simulink model "AccTarSel"  (R2018b)
settings: Solver=FixedStepDiscrete  StartTime=0.0  StopTime=inf  FixedStep=0.01  RelTol=1e-3
PostLoadFcn:
  | if any(exist('dsrtsu_mdlpostloadfcn', 'file') ~= 0), dsrtsu_mdlpostloadfcn('Execute', bdroot); end
values from neighbouring files (symbols this model uses):
  P_adtMaxBDC = 1.0    [AccTarSel.sldd]
  P_aFOCApproachIntpAcitve = -0.6    [AccTarSel.sldd]
  P_aFOCApproachIntpEnsure = -1.8    [AccTarSel.sldd]
  P_CutInEnable = 1.0    [AccTarSel.sldd]
  P_dAimMin = 4.5    [AccTarSel.sldd]
  P_dAimMinAVP = 1.5    [AccTarSel.sldd]
  P_dObjDrvOffMax = 5.0    [AccTarSel.sldd]
  P_dObjDrvOffMin = 3.0    [AccTarSel.sldd]
  P_dObjLowHystDecToStop = 4.5    [AccTarSel.sldd]
  P_dObjLowHystDecToStopAVP = 1.5    [AccTarSel.sldd]
  P_dObjUpperHystDecToStop = 5.0    [AccTarSel.sldd]
  P_dResMax = 5.0    [AccTarSel.sldd]
  P_dStandStill = 3.0    [AccTarSel.sldd]
  P_dStandStillMin = 2.0    [AccTarSel.sldd]
  P_dvarYMax4PO = 1.0    [AccTarSel.sldd]
  P_dyCutInThres = 3.6    [AccTarSel.sldd]
  P_facBDCInit = 0.7    [AccTarSel.sldd]
  P_facBDCIterCalc = 0.8    [AccTarSel.sldd]
  P_facFOCNegDiff = 0.3    [AccTarSel.sldd]
  P_facFOCPosDiff = 0.2    [AccTarSel.sldd]
  P_kapHystThres = 0.0005    [AccTarSel.sldd]
  P_PlausIntegDisable = 0.0    [AccTarSel.sldd]
  P_plausMin4PO = 0.5    [AccTarSel.sldd]
  P_probExistMin4PO = 0.8    [AccTarSel.sldd]
  P_StandObjEnable = 0.0    [AccTarSel.sldd]
  P_tAxTrackNegLower = 0.3    [AccTarSel.sldd]
  P_tAxTrackNegUpper = 0.6    [AccTarSel.sldd]
  P_tAxTrackPosLower = 1.0    [AccTarSel.sldd]
  P_tAxTrackPosUpper = 2.0    [AccTarSel.sldd]
  P_tBDCStartFilt = 0.2    [AccTarSel.sldd]
  P_tCSC = 3.5    [AccTarSel.sldd]
  P_tCurvFilt = 0.2    [AccTarSel.sldd]
  P_tCutInFilt = 0.5    [AccTarSel.sldd]
  P_tFiltAxAbsPONegFast = 0.1    [AccTarSel.sldd]
  P_tFiltAxAbsPONegSlow = 0.4    [AccTarSel.sldd]
  P_tFiltAxAbsPOPosFast = 1.2    [AccTarSel.sldd]
  P_tFiltAxAbsPOPosSlow = 2.0    [AccTarSel.sldd]
  P_tFiltAxAbsPOStand = 2.0    [AccTarSel.sldd]
  P_tFiltDAim = 0.1    [AccTarSel.sldd]
  P_tFiltDsd = 0.1    [AccTarSel.sldd]
  P_tFiltSpdLim = 3.0    [AccTarSel.sldd]
  P_tFiltVxAxPOFast = 0.15    [AccTarSel.sldd]
  P_tFiltVxAxPOSlow = 0.25    [AccTarSel.sldd]
  P_tFOCStatAccelFast = 4.0    [AccTarSel.sldd]
  P_tFOCStatAccelSlow = 3.5    [AccTarSel.sldd]
  P_tFOCStatDecelFast = 4.0    [AccTarSel.sldd]
  P_tFOCStatDecelSlow = 3.2    [AccTarSel.sldd]
  P_tMinDrvPhase = 2.0    [AccTarSel.sldd]
  P_tPredObjLeav = 1.2    [AccTarSel.sldd]
  P_tRollingFilt = 0.5    [AccTarSel.sldd]
  P_tRollingFinFilt = 1.0    [AccTarSel.sldd]
  P_tSSCNeg = 4.5    [AccTarSel.sldd]
  P_tSSCPos = 5.5    [AccTarSel.sldd]
  P_tToStop = 5.0    [AccTarSel.sldd]
  P_tToStopInBDC = 6.0    [AccTarSel.sldd]
  P_tToStopTrig = 4.0    [AccTarSel.sldd]
  P_vEgoDecToStop = 3.0    [AccTarSel.sldd]
  P_vEgoLowBDC = 4.0    [AccTarSel.sldd]
  P_vFOCNegDiff = 4.0    [AccTarSel.sldd]
  P_vFOCPosDiff = 5.0    [AccTarSel.sldd]
  P_vFOCStationaryFast = 15.0    [AccTarSel.sldd]
  P_vFOCStationarySlow = 5.0    [AccTarSel.sldd]
  P_vObjDrvOff = 0.5    [AccTarSel.sldd]
  P_vObjLowHystDecToStop = 0.5    [AccTarSel.sldd]
  P_vObjNoStop = 1.0    [AccTarSel.sldd]
  P_vObjReCalc = 1.0    [AccTarSel.sldd]
  P_vObjStop = 0.3    [AccTarSel.sldd]
  P_vObjUpperHystDecToStop = 0.8    [AccTarSel.sldd]
  P_vStandStill = 0.3    [AccTarSel.sldd]
  P_vStandStillHyst = 0.3    [AccTarSel.sldd]
  P_vyCutInThres = 0.5    [AccTarSel.sldd]
libraries: simulink x21, LPFilter x12
(part 4 of 11)

== system AccTarSel/ACC_dTarSet1/If Action Subsystem2 ==
  In1 : Inport
  Action Port : ActionPort  ActionType=else
  Out1 : Outport
  wires:
  In1/1 -> Out1/1

== system AccTarSel/ACC_dTarSet1/Subsystem ==
  ACCState : Inport
  Constant : Constant  Value=2  OutDataTypeStr=single
  Equal1 : RelationalOperator  Operator===  OutDataTypeStr=boolean  RndMeth=Simplest
  PreCon : Outport
  wires:
  Constant/1 -> Equal1/2
  ACCState/1 -> Equal1/1
  Equal1/1 -> PreCon/1

== system AccTarSel/AVP_Simu/AVP_Activate ==
  Action Port : ActionPort  ActionType=then
  Constant : Constant  OutDataTypeStr=single
  Out1 : Outport
  wires:
  Constant/1 -> Out1/1

== system AccTarSel/AVP_Simu/AVP_Deactivate ==
  Action Port : ActionPort  ActionType=elseif
  Constant : Constant  Value=0  OutDataTypeStr=single
  Out1 : Outport
  wires:
  Constant/1 -> Out1/1

== system AccTarSel/AVP_Simu/Hold ==
  AVP_ActiveK1 : Inport
  Action Port : ActionPort  ActionType=else
  Out1 : Outport
  wires:
  AVP_ActiveK1/1 -> Out1/1

== system AccTarSel/AVP_Simu/calcAVPInfo ==
  note: 00: Invalid
      | 01:Parking In
      | 02:Parking Out
      | 03:Stop
  AVP_Info : Inport
  egoInfo : Inport  Port=2
  SYS_Info : Inport  Port=3
  Bus Creator : BusCreator  Inputs=7  OutDataTypeStr=Bus: AVP_OUTPUT_ST  NonVirtualBus=on
      settings: InheritFromInputs=off
  Bus Selector : BusSelector  OutputSignals=EndPoint_x,AVP_STATE
  Traj_C{0..3} (4 alike) : Constant  Value=0  OutDataTypeStr=single
  dxPredict : Subsystem
  dy : Constant  Value=0  OutDataTypeStr=single
  Out1 : Outport
  wires:
  egoInfo/1 -> dxPredict/2(egoInfo)
  Traj_C1/1 -> Bus Creator/2
  Traj_C2/1 -> Bus Creator/3
  Traj_C3/1 -> Bus Creator/4
  Bus Selector/2 -> Bus Creator/7  "<AVP_STATE>"
  SYS_Info/1 -> dxPredict/3(SYS_Info)
  Traj_C0/1 -> Bus Creator/1
  dxPredict/1(dxPredict) -> Bus Creator/5
  dy/1 -> Bus Creator/6
  Bus Selector/1 -> dxPredict/1(dxSet)  "<EndPoint_x>"
  Bus Creator/1 -> Out1/1
  AVP_Info/1 -> Bus Selector/1

== system AccTarSel/AVP_Simu/default ==
  note: 00: Invalid
      | 01:Parking In
      | 02:Parking Out
      | 03:Stop
  AVP_State : Constant  Value=0  OutDataTypeStr=uint8
  Bus Creator : BusCreator  Inputs=7  OutDataTypeStr=Bus: AVP_OUTPUT_ST  NonVirtualBus=on
      settings: InheritFromInputs=off
  Traj_C{0..3} (4 alike) : Constant  Value=0  OutDataTypeStr=single
  dx : Constant  Value=255  OutDataTypeStr=single
  dy : Constant  Value=0  OutDataTypeStr=single
  Out1 : Outport
  wires:
  Bus Creator/1 -> Out1/1
  dy/1 -> Bus Creator/6
  dx/1 -> Bus Creator/5
  Traj_C0/1 -> Bus Creator/1
  Traj_C3/1 -> Bus Creator/4
  Traj_C2/1 -> Bus Creator/3
  Traj_C1/1 -> Bus Creator/2
  AVP_State/1 -> Bus Creator/7

== system AccTarSel/EgoCourseFusion/CurvatureFilt ==
  In1 : Inport
  In2 : Inport  Port=2
  1-D Lookup Table : Lookup_n-D  NumberOfTableDimensions=1  LookupTableObject=''  BreakpointsForDimension1=[-0.1,-0.0015,-0.0005,0.0005,0.0015,0.1]  BreakpointsForDimension1FirstPoint=10  BreakpointsForDimension2FirstPoint=10  BreakpointsForDimension1Spacing=12  BreakpointsForDimension2Spacing=12  IndexSearchMethod=Linear search  Table=[-0.1,-0.0015,0,0,0.0015,0.1]  InternalRulePriority=Speed  RndMeth=Simplest  InputSameDT=on
  Abs : Abs
  Add : Sum  Inputs=+-
  Add1 : Sum
  Constant1 : Constant  Value=0  OutDataTypeStr=single
  Constant3 : Constant  OutDataTypeStr=single
  Divide : Product  Inputs=*/
  If : If  IfExpression=u1 == 1
  If Action Subsystem : Subsystem  TreatAsAtomicUnit=on
  If Action Subsystem1 : Subsystem  TreatAsAtomicUnit=on
  Memory : Memory
  Merge : Merge
  Multiply : Product
  Multiply1 : Product
  P_kapHystThres : Constant  Value=P_kapHystThres
  P_tCurvFilt : Constant  Value=P_tCurvFilt
  Relational Operator : RelationalOperator  Operator=<=  OutDataTypeStr=boolean  RndMeth=Simplest
  To Workspace : ToWorkspace  VariableName=kapHyst  SaveFormat=Timeseries  SampleTime=-1
  kapTrajFilt : Outport
  wires:
  In1/1 -> 1-D Lookup Table/1, Abs/1
  P_kapHystThres/1 -> Relational Operator/2
  Abs/1 -> Relational Operator/1
  Relational Operator/1 -> If/1
  Constant1/1 -> If Action Subsystem/1(In1)
  If/1 -> If Action Subsystem/Action
  If/2 -> If Action Subsystem1/Action
  1-D Lookup Table/1 -> If Action Subsystem1/1(In1)
  If Action Subsystem/1(Out1) -> Merge/1
  If Action Subsystem1/1(Out1) -> Merge/2
  P_tCurvFilt/1 -> Divide/2
  In2/1 -> Divide/1
  Merge/1 -> To Workspace/1, Multiply/1
  Divide/1 -> Add/2, Multiply/2
  Multiply/1 -> Add1/1
  Memory/1 -> Multiply1/2
  Multiply1/1 -> Add1/2
  Add1/1 -> kapTrajFilt/1, Memory/1
  Constant3/1 -> Add/1
  Add/1 -> Multiply1/1

== system AccTarSel/ObjAdapter/For Each Subsystem ==
  note: Type:
      | 0	Unknown
      | 1	Pedestrain
      | 2	Bi/Motor cycle
      | >=3	Vehicle
  note: MotionSts:
      | 0	Unknown
      | 1	Standstill
      | 2	Driving
      | 3	InvDriving
      | 4	Stopped
      | 5	InvStopped
  In1 : Inport  Partition=on  PartitionDimension=1  PartitionWidth=1  PartitionOffset=0
  In2 : Inport  Port=2
  Add : Sum  Inputs=+-
  Add1 : Sum  Inputs=+-
  Bus Creator : BusCreator  Inputs=14  OutDataTypeStr=Bus: OBJDATA_ST  NonVirtualBus=on
      settings: InheritFromInputs=off
  Bus Selector : BusSelector  OutputSignals=obj_property.trackStatus,obj_information.valid,obj_estimate.longPosition,obj_information.length,obj_estimate.latPosition,obj_estimate.longAbsoluteVelocity,obj_estimate.latRelativeVelocity,obj_estimate.longAbsoluteAcceleration,obj_estimate.latRelativeAcceleration,obj_information.motionPatternCurrent,obj_information.type,obj_property.id
  Bus Selector1 : BusSelector  OutputSignals=vRef,aRef
  Constant1 : Constant  Value=0  OutDataTypeStr=single
  Constant2 : Constant  Value=0  OutDataTypeStr=single
  Constant3 : Constant  Value=0.999  OutDataTypeStr=single
  Data Type Conversion : DataTypeConversion  OutDataTypeStr=boolean
  Data Type Conversion{2..3,5..8} (6 alike) : DataTypeConversion
  For Each : ForEach  DisableCoverage=on  IndexMode=One-based
  calcDx : Subsystem
  calcHist : Subsystem
  Out1 : Outport  OutDataTypeStr=Bus: OBJDATA_ST  ConcatenationDimension=1
  wires:
  In1/1 -> Bus Selector/1
  Bus Creator/1 -> Out1/1
  Bus Selector/2 -> Data Type Conversion/1  "<valid>"
  Data Type Conversion/1 -> Bus Creator/2  "Valid"
  Constant1/1 -> Bus Creator/4  "dvarX"
  Constant2/1 -> Bus Creator/6  "dvarY"
  Data Type Conversion2/1 -> Bus Creator/5  "dy"
  Bus Selector/1 -> calcHist/1(<trackStatus>)  "<trackStatus>"
  calcHist/1(Hist) -> Bus Creator/1
  Bus Selector/3 -> calcDx/1(<longPosition>)  "<longPosition>"
  Bus Selector/4 -> calcDx/2(<length>)  "<length>"
  calcDx/1(dx) -> Bus Creator/3
  Bus Selector/5 -> Data Type Conversion2/1  "<latPosition>"
  Add/1 -> Bus Creator/7  "vx"
  Bus Selector/7 -> Data Type Conversion3/1  "<latRelativeVelocity>"
  Data Type Conversion3/1 -> Bus Creator/8  "vy"
  Add1/1 -> Bus Creator/9  "ax"
  Bus Selector/9 -> Data Type Conversion5/1  "<latRelativeAcceleration>"
  Data Type Conversion5/1 -> Bus Creator/10  "ay"
  Bus Selector/10 -> Data Type Conversion6/1  "<motionPatternCurrent>"
  Data Type Conversion6/1 -> Bus Creator/11  "MotionSts"
  Bus Selector/11 -> Data Type Conversion7/1  "<type>"
  Data Type Conversion7/1 -> Bus Creator/12  "Type"
  Constant3/1 -> Bus Creator/13  "probExist"
  Bus Selector/12 -> Data Type Conversion8/1  "<id>"
  Data Type Conversion8/1 -> Bus Creator/14  "ID"
  In2/1 -> Bus Selector1/1
  Bus Selector1/1 -> [vRef]  "<vRef>"
  Bus Selector/6 -> Add/1  "<longAbsoluteVelocity>"
  [vRef] -> Add/2
  Bus Selector/8 -> Add1/1  "<longAbsoluteAcceleration>"
  Bus Selector1/2 -> [aRef]  "<aRef>"
  [aRef] -> Add1/2

== system AccTarSel/ObjRadarAdapter/For Each Subsystem ==
  In1 : Inport  Partition=on  PartitionDimension=1  PartitionWidth=1  PartitionOffset=0
  Bus Creator : BusCreator  Inputs=14  OutDataTypeStr=Bus: OBJDATA_ST  NonVirtualBus=on
  Bus Selector : BusSelector  OutputSignals=Obj_UpdateFlag,Obj_ValidFlag,Obj_XPos,Obj_YPos,Obj_XVelRel,Obj_YVelRel,Obj_XAccRel,Obj_MotionPattern,Obj_Type,Obj_ExstProb,Obj_ID
  Constant1 : Constant  Value=0  OutDataTypeStr=single
  Constant2 : Constant  Value=0  OutDataTypeStr=single
  Constant3 : Constant  Value=0.999  OutDataTypeStr=single
  Constant4 : Constant  Value=0  OutDataTypeStr=single
  Data Type Conversion : DataTypeConversion  OutDataTypeStr=boolean
  Data Type Conversion{1..4,6..8} (7 alike) : DataTypeConversion
  Data Type Conversion9 : DataTypeConversion  OutDataTypeStr=boolean
  For Each : ForEach  DisableCoverage=on  IndexMode=One-based
  Terminator : Terminator
  calcDx : Subsystem
  calcMotionSts : Subsystem
  calcType : Subsystem
  Out1 : Outport  ConcatenationDimension=1
  wires:
  In1/1 -> Bus Selector/1
  Constant3/1 -> Bus Creator/13  "probExist"
  Data Type Conversion/1 -> Bus Creator/2  "Valid"
  calcDx/1(dx) -> Bus Creator/3
  Data Type Conversion7/1 -> Bus Creator/12  "Type"
  Data Type Conversion3/1 -> Bus Creator/8  "vy"
  Constant4/1 -> Bus Creator/10  "ay"
  Data Type Conversion1/1 -> Bus Creator/7  "vx"
  Data Type Conversion4/1 -> Bus Creator/9  "ax"
  Data Type Conversion8/1 -> Bus Creator/14  "ID"
  Constant2/1 -> Bus Creator/6  "dvarY"
  Constant1/1 -> Bus Creator/4  "dvarX"
  Data Type Conversion6/1 -> Bus Creator/11  "MotionSts"
  Data Type Conversion2/1 -> Bus Creator/5  "dy"
  Data Type Conversion9/1 -> Bus Creator/1
  Bus Creator/1 -> Out1/1
  Bus Selector/1 -> Data Type Conversion9/1  "<Obj_UpdateFlag>"
  Bus Selector/2 -> Data Type Conversion/1  "<Obj_ValidFlag>"
  Bus Selector/3 -> calcDx/1(<longPosition>)  "<Obj_XPos>"
  Bus Selector/4 -> Data Type Conversion2/1  "<Obj_YPos>"
  Bus Selector/5 -> Data Type Conversion1/1  "<Obj_XVelRel>"
  Bus Selector/6 -> Data Type Conversion3/1  "<Obj_YVelRel>"
  Bus Selector/7 -> Data Type Conversion4/1  "<Obj_XAccRel>"
  Bus Selector/8 -> calcMotionSts/1(MotionPattern)  "<Obj_MotionPattern>"
  calcMotionSts/1(MotionSts) -> Data Type Conversion6/1
  Bus Selector/9 -> calcType/1(ObjType)  "<Obj_Type>"
  calcType/1(Type) -> Data Type Conversion7/1
  Bus Selector/10 -> Terminator/1  "<Obj_ExstProb>"
  Bus Selector/11 -> Data Type Conversion8/1  "<Obj_ID>"

== system AccTarSel/RTI Data/RTI Data Store ==
  RTI Data Store : Subsystem  mask(RTI_DATA_STORE){}
      mask help:
      | RTI Data Store Block. This block is used by RTI to store internal model dependent data. Deleting this block will result in data loss.
      |
      | NEVER DELETE, COPY, OR MODIFY THIS BLOCK!
      mask Help:
      | RTI Data Store Block. This block is used by RTI to store internal model dependent data. Deleting this block will result in data loss.
      | 
      | NEVER DELETE, COPY, OR MODIFY THIS BLOCK!
      mask Display: text(0.5, 0.5, ' ', 'HorizontalAlignment', 'center');

== system AccTarSel/Subsystem1/If Action Subsystem ==
  In1 : Inport
  Action Port : ActionPort  ActionType=then
  Out1 : Outport
  wires:
  In1/1 -> Out1/1

== system AccTarSel/Subsystem1/If Action Subsystem1 ==
  In1 : Inport
  Action Port : ActionPort  ActionType=else
  Out1 : Outport
  wires:
  In1/1 -> Out1/1

== system AccTarSel/Subsystem3/calcOverride ==
  VLC_Cmd_K1 : Inport
  AccelPedal : Inport  Port=2
  PTOverride : Inport  Port=3
  AND : Logic  Inputs=3  AllPortsSameDT=off  OutDataTypeStr=boolean
  AND1 : Logic  Operator=OR  AllPortsSameDT=off  OutDataTypeStr=boolean
  AND2 : Logic  Inputs=3  AllPortsSameDT=off  OutDataTypeStr=boolean
  AND3 : Logic  Operator=OR  AllPortsSameDT=off  OutDataTypeStr=boolean
  AND4 : Logic  Operator=NOT  AllPortsSameDT=off  OutDataTypeStr=boolean
  Bus Selector : BusSelector  OutputSignals=CDDEnable
  Constant : Constant  Value=15
  Constant1 : Constant  Value=10
  Memory : Memory
  Relational Operator : RelationalOperator  OutDataTypeStr=boolean  RndMeth=Simplest
  Relational Operator1 : RelationalOperator  OutDataTypeStr=boolean  RndMeth=Simplest
  DrvOverride : Outport
  wires:
  VLC_Cmd_K1/1 -> Bus Selector/1
  AccelPedal/1 -> Relational Operator1/1, Relational Operator/1
  Constant/1 -> Relational Operator/2
  Bus Selector/1 -> AND/2  "<CDDEnable>"
  Relational Operator/1 -> AND/3
  AND3/1 -> AND1/1, Memory/1
  PTOverride/1 -> AND4/1, AND1/2
  AND1/1 -> DrvOverride/1
  Memory/1 -> AND2/3
  AND/1 -> AND3/1
  AND2/1 -> AND3/2
  Constant1/1 -> Relational Operator1/2
  Relational Operator1/1 -> AND2/1
  AND4/1 -> AND2/2, AND/1

== system AccTarSel/Target_PreProcess/AVP_Target ==
  note: 00: Invalid
      | 01:Parking In
      | 02:Parking Out
      | 03:Stop
  AVP_Info : Inport
  vRef : Inport  Port=2
  aRef : Inport  Port=3
  Bus Selector : BusSelector  OutputSignals=AVP_STATE
  Constant : Constant  Value=0  OutDataTypeStr=uint8
  If : If  IfExpression=u1 == 1
  If Action Subsystem : Subsystem  TreatAsAtomicUnit=on
  If Action Subsystem1 : Subsystem  TreatAsAtomicUnit=on
  Merge : Merge
  Relational Operator : RelationalOperator  Operator=>  OutDataTypeStr=boolean  RndMeth=Simplest
  AVP_Target : Outport
  wires:
  vRef/1 -> If Action Subsystem/2(vRef)
  aRef/1 -> If Action Subsystem/3(aRef)
  If/1 -> If Action Subsystem/Action
  If/2 -> If Action Subsystem1/Action
  If Action Subsystem/1(Virtual_Object) -> Merge/1
  If Action Subsystem1/1(Default) -> Merge/2
  Merge/1 -> AVP_Target/1
  AVP_Info/1 -> If Action Subsystem/1(AVP_Info), Bus Selector/1
  Bus Selector/1 -> Relational Operator/1  "<AVP_STATE>"
  Constant/1 -> Relational Operator/2
  Relational Operator/1 -> If/1

== system AccTarSel/Target_PreProcess/If Action Subsystem ==
  dx : Inport
  vx : Inport  Port=2
  ax : Inport  Port=3
  aRef : Inport  Port=4
  Action Port : ActionPort  ActionType=else
  Add : Sum
  Constant : Constant  Value=0  OutDataTypeStr=single
  dxPreFiltInit : Outport
  vxPreFiltInit : Outport  Port=2
  axPreFiltInit : Outport  Port=3
  axAbsPreFiltInit : Outport  Port=4
  NegTimeInit : Outport  Port=5
  PosTimeInit : Outport  Port=6
  wires:
  vx/1 -> vxPreFiltInit/1
  ax/1 -> Add/1, axPreFiltInit/1
  aRef/1 -> Add/2
  Add/1 -> axAbsPreFiltInit/1
  dx/1 -> dxPreFiltInit/1
  Constant/1 -> PosTimeInit/1, NegTimeInit/1

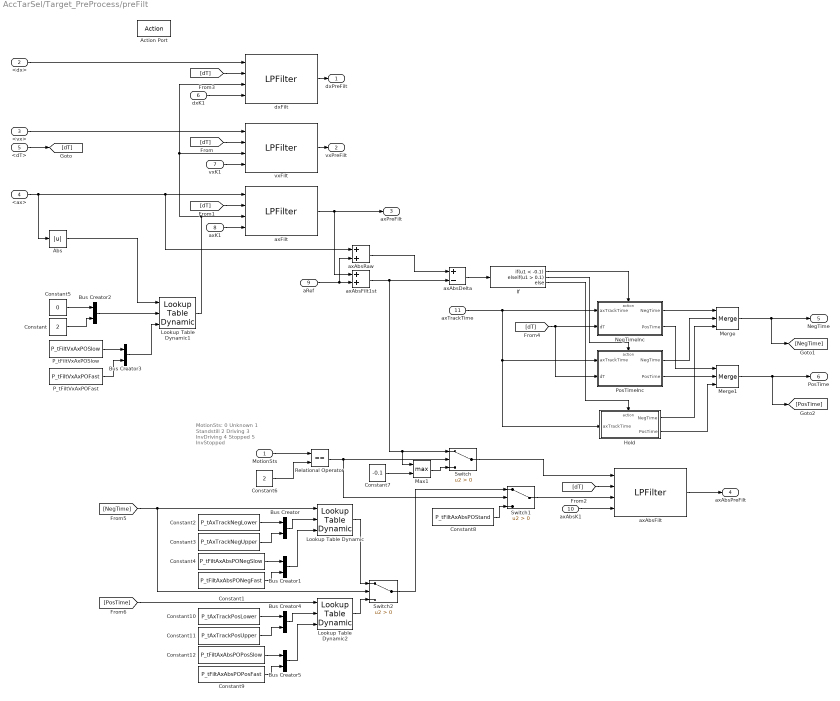
== system AccTarSel/Target_PreProcess/preFilt ==
  note: MotionSts:
      | 0	Unknown
      | 1	Standstill
      | 2	Driving
      | 3	InvDriving
      | 4	Stopped
      | 5	InvStopped
  MotionSts : Inport
  <dx> : Inport  Port=2
  <vx> : Inport  Port=3
  <ax> : Inport  Port=4
  <dT> : Inport  Port=5
  dxK1 : Inport  Port=6
  vxK1 : Inport  Port=7
  axK1 : Inport  Port=8
  aRef : Inport  Port=9
  axAbsK1 : Inport  Port=10
  axTrackTime : Inport  Port=11
  Action Port : ActionPort  ActionType=then
  Abs : Abs
  Bus Creator{,1..5} (6 alike) : BusCreator  Inputs=2
  Constant : Constant  Value=2  OutDataTypeStr=single
  Constant1 : Constant  Value=P_tFiltAxAbsPONegFast
  Constant10 : Constant  Value=P_tAxTrackPosLower
  Constant11 : Constant  Value=P_tAxTrackPosUpper
  Constant12 : Constant  Value=P_tFiltAxAbsPOPosSlow
  Constant2 : Constant  Value=P_tAxTrackNegLower
  Constant3 : Constant  Value=P_tAxTrackNegUpper
  Constant4 : Constant  Value=P_tFiltAxAbsPONegSlow
  Constant5 : Constant  Value=0  OutDataTypeStr=single
  Constant6 : Constant  Value=2  OutDataTypeStr=single
  Constant7 : Constant  Value=-0.1  OutDataTypeStr=single
  Constant8 : Constant  Value=P_tFiltAxAbsPOStand
  Constant9 : Constant  Value=P_tFiltAxAbsPOPosFast
  Hold : Subsystem  TreatAsAtomicUnit=on
  If : If  IfExpression=u1 < -0.1  ElseIfExpressions=u1 > 0.1
  Lookup Table Dynamic : simulink/Lookup Tables/Lookup Table Dynamic  LookUpMeth=Interpolation-Use End Values  OutDataType=fixdt('single')  OutScaling=[]  OutputDataTypeScalingMode=Specify via dialog  OutDataTypeStr=single  DoSatur=off
      settings: SourceProductName=Simulink
  Lookup Table Dynamic1 : simulink/Lookup Tables/Lookup Table Dynamic  LookUpMeth=Interpolation-Use End Values  OutDataType=fixdt('single')  OutScaling=[]  OutputDataTypeScalingMode=Specify via dialog  OutDataTypeStr=single  DoSatur=off
      settings: SourceProductName=Simulink
  Lookup Table Dynamic2 : simulink/Lookup Tables/Lookup Table Dynamic  LookUpMeth=Interpolation-Use End Values  OutDataType=fixdt('single')  OutScaling=[]  OutputDataTypeScalingMode=Specify via dialog  OutDataTypeStr=single  DoSatur=off
      settings: SourceProductName=Simulink
  Max1 : MinMax  Function=max  Inputs=2
  Merge : Merge  Inputs=3
  Merge1 : Merge  Inputs=3
  NegTimeInc : Subsystem  TreatAsAtomicUnit=on
  P_tFiltVxAxPOFast : Constant  Value=P_tFiltVxAxPOFast
  P_tFiltVxAxPOSlow : Constant  Value=P_tFiltVxAxPOSlow
  PosTimeInc : Subsystem  TreatAsAtomicUnit=on
  Relational Operator : RelationalOperator  Operator===  OutDataTypeStr=boolean  RndMeth=Simplest
  Switch : Switch  Criteria=u2 > Threshold
  Switch1 : Switch  Criteria=u2 > Threshold
  Switch2 : Switch  Criteria=u2 > Threshold
  axAbsDelta : Sum  Inputs=+-
  axAbsFilt : LPFilter/LPFilter  SystemSampleTime=-1
      settings: SourceProductName=CustomLib
  axAbsFilt1st : Sum
  axAbsRaw : Sum
  axFilt : LPFilter/LPFilter  SystemSampleTime=-1
      settings: SourceProductName=CustomLib
  dxFilt : LPFilter/LPFilter  SystemSampleTime=-1
      settings: SourceProductName=CustomLib
  vxFilt : LPFilter/LPFilter  SystemSampleTime=-1
      settings: SourceProductName=CustomLib
  dxPreFilt : Outport
  vxPreFilt : Outport  Port=2
  axPreFilt : Outport  Port=3
  axAbsPreFilt : Outport  Port=4
  NegTime : Outport  Port=5
  PosTime : Outport  Port=6
  wires:
  axK1/1 -> axFilt/4
  axFilt/1 -> axAbsFilt1st/1, axPreFilt/1
  vxFilt/1 -> vxPreFilt/1
  <ax>/1 -> axAbsRaw/1, axFilt/1, Abs/1
  <vx>/1 -> vxFilt/1
  vxK1/1 -> vxFilt/4
  aRef/1 -> axAbsRaw/2, axAbsFilt1st/2
  axAbsFilt1st/1 -> Max1/1, Switch/1, axAbsDelta/2
  axAbsK1/1 -> axAbsFilt/4
  axAbsFilt/1 -> axAbsPreFilt/1
  <dT>/1 -> [dT]
  [dT] -> vxFilt/2
  [dT] -> axFilt/2
  [dT] -> axAbsFilt/2
  Lookup Table Dynamic1/1 -> dxFilt/3, vxFilt/3, axFilt/3
  <dx>/1 -> dxFilt/1
  [dT] -> dxFilt/2
  dxK1/1 -> dxFilt/4
  dxFilt/1 -> dxPreFilt/1
  axAbsDelta/1 -> If/1
  Constant2/1 -> Bus Creator/1
  Constant3/1 -> Bus Creator/2
  Bus Creator/1 -> Lookup Table Dynamic/2
  Lookup Table Dynamic/1 -> Switch2/1
  Bus Creator1/1 -> Lookup Table Dynamic/3
  Constant5/1 -> Bus Creator2/1
  Constant/1 -> Bus Creator2/2
  Bus Creator2/1 -> Lookup Table Dynamic1/2
  P_tFiltVxAxPOSlow/1 -> Bus Creator3/1
  P_tFiltVxAxPOFast/1 -> Bus Creator3/2
  Bus Creator3/1 -> Lookup Table Dynamic1/3
  Abs/1 -> Lookup Table Dynamic1/1
  axAbsRaw/1 -> axAbsDelta/1
  axTrackTime/1 -> PosTimeInc/1(axTrackTime), Hold/1(axTrackTime), NegTimeInc/1(axTrackTime)
  If/1 -> NegTimeInc/Action
  If/2 -> PosTimeInc/Action
  If/3 -> Hold/Action
  [dT] -> NegTimeInc/2(dT), PosTimeInc/2(dT)
  NegTimeInc/1(NegTime) -> Merge/1
  PosTimeInc/1(NegTime) -> Merge/2
  Hold/1(NegTime) -> Merge/3
  PosTimeInc/2(PosTime) -> Merge1/2
  NegTimeInc/2(PosTime) -> Merge1/1
  Hold/2(PosTime) -> Merge1/3
  Merge1/1 -> [PosTime], PosTime/1
  Merge/1 -> [NegTime], NegTime/1
  Constant4/1 -> Bus Creator1/1
  Constant1/1 -> Bus Creator1/2
  MotionSts/1 -> Relational Operator/1
  Constant6/1 -> Relational Operator/2
  Relational Operator/1 -> Switch/2, Switch1/2
  Switch/1 -> axAbsFilt/1
  Switch1/1 -> axAbsFilt/3
  Constant7/1 -> Max1/2
  Max1/1 -> Switch/3
  Constant8/1 -> Switch1/3
  [NegTime] -> Switch2/2, Lookup Table Dynamic/1
  Constant9/1 -> Bus Creator5/2
  Constant12/1 -> Bus Creator5/1
  Bus Creator5/1 -> Lookup Table Dynamic2/3
  Bus Creator4/1 -> Lookup Table Dynamic2/2
  Constant11/1 -> Bus Creator4/2
  Constant10/1 -> Bus Creator4/1
  [PosTime] -> Lookup Table Dynamic2/1
  Lookup Table Dynamic2/1 -> Switch2/3
  Switch2/1 -> Switch1/1

== system AccTarSel/calcCancelFlag/If Action Subsystem ==
  Action Port : ActionPort  ActionType=then
  Constant : Constant  OutDataTypeStr=boolean
  Constant1 : Constant  Value=0.5  OutDataTypeStr=single
  CancelFlag : Outport
  HoldTime : Outport  Port=2
  wires:
  Constant/1 -> CancelFlag/1
  Constant1/1 -> HoldTime/1
